simulink model "finalProjectLQGLinearized"  (R2015b)
settings: Solver=VariableStepAuto  StartTime=0.0  StopTime=50  RelTol=1e-3
undefined symbols (not defined in the file): A1, B1, C, Continuous, K, Nbar, Time, X0
libraries: ctrlSharedLib x1
settings Model: Creator=Rishabh  LastModifiedBy=rbiyani
settings DataIOCC: LimitDataPoints=off
settings DebuggingCC: AllowSymbolicDim=on
settings ModelReferenceCC: PropagateSignalLabelsOutOfModel=on
settings GRTTargetCC: GeneratePreprocessorConditionals=Disable all

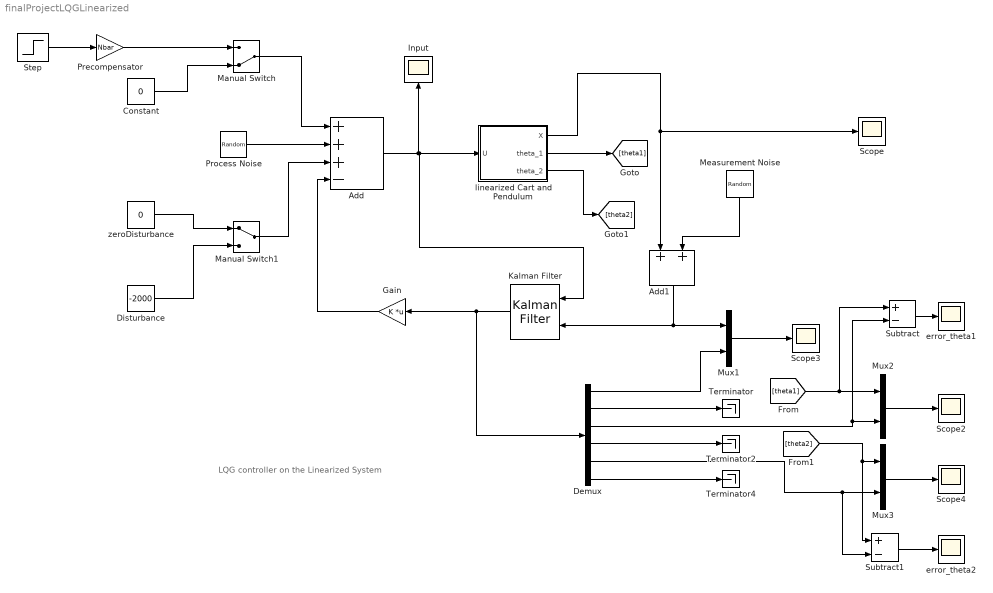
== system finalProjectLQGLinearized ==
  note: LQG controller on the Linearized System
  Add : Sum  Inputs=+++-
  Add1 : Sum
  Constant : Constant  Value=0
  Demux : Demux  Outputs=6
  Disturbance : Constant  Value=-2000
  Gain : Gain  Gain=K  Multiplication=Matrix(K*u)
  Input : Scope
  Kalman Filter : ctrlSharedLib/Kalman Filter  TimeDomain=Continuous-Time  UseCurrentEstimator=on  ModelSource=Individual A, B, C, D matrices  ModelSourceVariable=ss(0.95,1,1,0,1)  A=A1  B=B1  C=C  D=0  NumberOfStates=1  NumberOfInputs=1  NumberOfOutputs=1  InitialEstimateSource=Dialog  X0=[0 0 X0(3) 0 X0(5) 0]  P0=10  UseK=off  UseGH=on  NumberOfProcessNoiseInputs=1  G=B1  TimeInvariantG=on  H=0  TimeInvariantH=on  Q=0.2  TimeInvariantQ=on  R=0.001  TimeInvariantR=on  N=0  TimeInvariantN=on  AddInputPort=on  AddEnablePort=off  OutputEstimatedY=off  OutputP=off  Ts=-1
  Manual Switch : ManualSwitch  CurrentSetting=0
  Manual Switch1 : ManualSwitch
  Measurement Noise : RandomNumber  Variance=0.001  SampleTime=0.1
  Mux1 : Mux  Inputs=2
  Mux2 : Mux  Inputs=2
  Mux3 : Mux  Inputs=2
  Precompensator : Gain  Gain=Nbar
  Process Noise : RandomNumber  Variance=0.2  SampleTime=0.1
  Scope{,2..4} (4 alike) : Scope
  Step : Step  After=10  SampleTime=0
  Subtract : Sum  Inputs=+-
  Subtract1 : Sum  Inputs=+-
  Terminator : Terminator
  Terminator2 : Terminator
  Terminator4 : Terminator
  error_theta1 : Scope
  error_theta2 : Scope
  "linearized Cart and Pendulum " : Subsystem
  zeroDisturbance : Constant  Value=0
  wires:
  "linearized Cart and Pendulum "/1(X) -> Add1/1, Scope/1
  Add1/1 -> Mux1/1, Kalman Filter/2
  Kalman Filter/1 -> Demux/1, Gain/1
  Demux/1 -> Mux1/2
  Mux1/1 -> Scope3/1
  Demux/2 -> Terminator/1
  Demux/4 -> Terminator2/1
  Demux/6 -> Terminator4/1
  Demux/3 -> Mux2/2, Subtract/2
  [theta1] -> Mux2/1, Subtract/1
  [theta2] -> Mux3/1, Subtract1/1
  Demux/5 -> Subtract1/2, Mux3/2
  Mux2/1 -> Scope2/1
  Mux3/1 -> Scope4/1
  Add/1 -> "linearized Cart and Pendulum "/1(U), Kalman Filter/1, Input/1
  "linearized Cart and Pendulum "/2(theta_1) -> [theta1]
  "linearized Cart and Pendulum "/3(theta_2) -> [theta2]
  Subtract/1 -> error_theta1/1
  Subtract1/1 -> error_theta2/1
  Step/1 -> Precompensator/1
  Constant/1 -> Manual Switch/2
  Manual Switch/1 -> Add/1
  Precompensator/1 -> Manual Switch/1
  Process Noise/1 -> Add/2
  Measurement Noise/1 -> Add1/2
  Gain/1 -> Add/4
  zeroDisturbance/1 -> Manual Switch1/1
  Disturbance/1 -> Manual Switch1/2
  Manual Switch1/1 -> Add/3

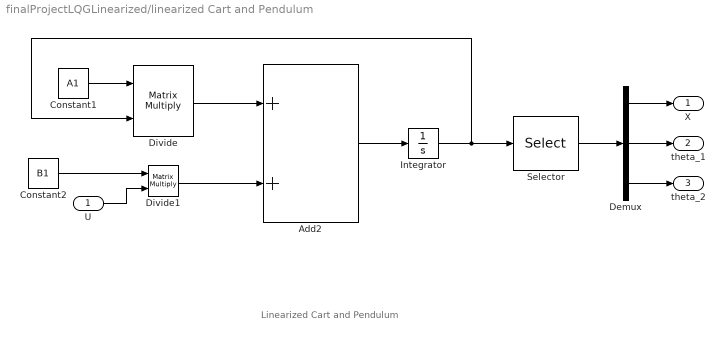
== system finalProjectLQGLinearized/linearized Cart and Pendulum  ==
  note: Linearized Cart and Pendulum
  U : Inport
  Add2 : Sum
  Constant1 : Constant  Value=A1
  Constant2 : Constant  Value=B1
  Demux : Demux  Outputs=3
  Divide : Product  Inputs=**  Multiplication=Matrix(*)
  Divide1 : Product  Inputs=**  Multiplication=Matrix(*)
  Integrator : Integrator  InitialCondition=X0
  Selector : Selector  InputPortWidth=6  IndexOptions=Index vector (dialog)  Indices=[1 3 5]  OutputSizes=1
  X : Outport
  theta_1 : Outport  Port=2
  theta_2 : Outport  Port=3
  wires:
  U/1 -> Divide1/2
  Divide1/1 -> Add2/2
  Add2/1 -> Integrator/1
  Constant2/1 -> Divide1/1
  Divide/1 -> Add2/1
  Constant1/1 -> Divide/1
  Integrator/1 -> Selector/1, Divide/2
  Selector/1 -> Demux/1
  Demux/3 -> theta_2/1
  Demux/2 -> theta_1/1
  Demux/1 -> X/1
